simulink model "week3_2"  (R2020b)
settings: Solver=VariableStepAuto  StartTime=0.0  StopTime=inf  RelTol=1e-3
settings Model: EnablePacing=on  PacingRate=0.100000  Creator=Lenovo  LastModifiedBy=Lenovo

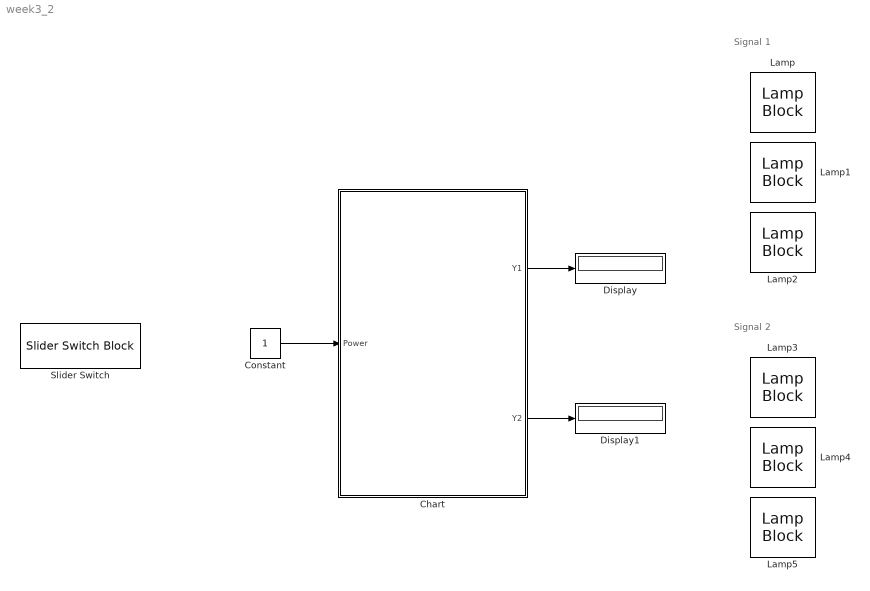
== system week3_2 ==
  note: Signal 1
  note: Signal 2
  Chart : Stateflow chart  TreatAsAtomicUnit=on
  Constant : Constant
  Display : Display
  Display1 : Display
  Lamp{,1..5} (6 alike) : LampBlock
  Slider Switch : SliderSwitchBlock
      settings: Values={{'Off', 'On'}, [0 1]}
  wires:
  Chart/2(Y2) -> Display1/1
  Chart/1(Y1) -> Display/1
  Constant/1 -> Chart/1(Power)

== stateflow chart week3_2/Chart ==
  state Signal_ON
    state Stop
      en:
      Y1=0;
      Y2=2;
    state Stop_1
      en:
      Y1=0;
      Y2=2;
    state Ready
      en:
      Y1=1;
      Y2=0;
    state Ready_1
      en:
      Y1=0;
      Y2=1;
    state GO
      en:
      Y1=2;
      Y2=0;
    (default) -> Stop
    Stop_1 -> Ready : {after(5,sec)}
    Stop -> Stop_1 : {after(3,sec)}
    Ready_1 -> Stop : {after(3,sec)}
    Ready -> GO : {after(3,sec)}
    GO -> Ready_1 : {after(5,sec)}
  state Signal_OFF
    en:
    Y1=1;
    Y2=1;
  (default) -> Signal_OFF
  Signal_OFF -> Signal_ON : [Power==1]
  Signal_ON -> Signal_OFF : [Power==0]
  data: Power input; Y1 output; Y2 output
